simulink model "CSE1_Full"  (R2019a)
settings: Solver=VariableStepAuto  StartTime=0.0  StopTime=200  MaxStep=10e-3  RelTol=1e-3
values from neighbouring files (symbols this model uses):
  alpha1 = 0    [main.m]
  alpha2 = 3*pi/4    (= 2.35619449019)    [main.m]
  b = [0;0;0]    [main.m]
  C1 = pinv(B1*K1)    [main.m]
  C2 = inv(K2)*inv(B2)    [main.m]
  center = [0; 0]    [main.m]
  D = [d_11 0 0 ... (first row only)    [main.m]
  inv_M = inv(M)    [main.m]
  K_1 = 10*diag([2 2 2])    [main.m]
  K_2 = 10*diag([2 2 2])    [main.m]
  L_1 = diag([12 12 12])    [main.m]
  L_2 = diag([8 8 8])    [main.m]
  L_3 = diag([1 1 1])    [main.m]
  M = [m_11 0    0 ... (first row only)    [main.m]
  mu = 10e-4    (= 0.001)    [main.m]
  pd_final = [10;4]    [main.m]
  pd_initial = [0;0]    [main.m]
  R = [2; 3]    [main.m]
  Umax_1 = 0.1    [main.m]
  Umax_2 = 0.05    [main.m]
libraries: lib x9
settings Model: Creator=einarsu  LastModifiedBy=zhy
settings DataIOCC: ReturnWorkspaceOutputs=off
settings DebuggingCC: PregeneratedLibrarySubsystemCodeDiagnostic=none  SFExecutionAtInitializationDiag=none  ArithmeticOperatorsInVariantConditions=warning
settings HardwareCC: TargetBitPerPointer=64  TargetBitPerSizeT=64  TargetBitPerPtrDiffT=64  TargetLongLongMode=on  TargetIntDivRoundTo=Zero  TargetEndianess=LittleEndian  TargetWordSize=64  TargetHWDeviceType=MATLAB Host  ProdEqTarget=off
settings SFSimCC: SimUseLocalCustomCode=off
settings RTWCC: SystemTargetFile=rsim.tlc  TemplateMakefile=rsim_default_tmf  Description=Rapid Simulation Target  RTWUseLocalCustomCode=off
settings CodeAppCC: StateflowObjectComments=on
settings TargetCC: TargetLangStandard=C99 (ISO)  ParMdlRefBuildCompliant=on  ConcurrentExecutionCompliant=on  GeneratePreprocessorConditionals=Use local settings  MatFileLogging=on  PreserveStateflowLocalDataDimensions=off

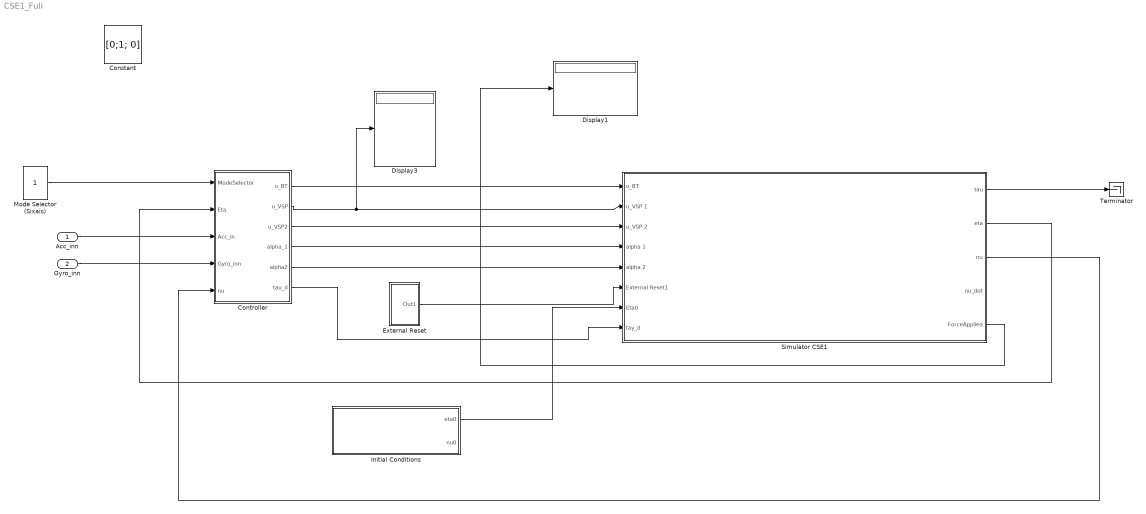
== system CSE1_Full ==
  Acc_inn : Inport
  Gyro_inn : Inport  Port=2
  Constant : Constant  Value=[0;1; 0]
  Controller : Subsystem
  Display1 : Display
  Display3 : Display
  External Reset : Subsystem
  "Initial Conditions " : Subsystem
  Mode Selector (Sixais) : Constant
  Simulator CSE1 : Subsystem
  Terminator : Terminator
  wires:
  Controller/1(u_BT) -> Simulator CSE1/1(u_BT)
  Controller/4(alpha_1) -> Simulator CSE1/4(alpha 1)
  Controller/2(u_VSP) -> Display3/1, Simulator CSE1/2(u_VSP 1)
  Controller/5(alpha2) -> Simulator CSE1/5(alpha 2)
  Controller/3("u_VSP2 ") -> Simulator CSE1/3(u_VSP 2)
  Simulator CSE1/1(tau) -> Terminator/1
  External Reset/1(Out1) -> Simulator CSE1/6(External Reset1)
  "Initial Conditions "/1(eta0) -> Simulator CSE1/7(Eta0)
  Mode Selector (Sixais)/1 -> Controller/1(ModeSelector)
  Simulator CSE1/2(eta) -> Controller/2(Eta)
  Acc_inn/1 -> Controller/3(Acc_in)
  Gyro_inn/1 -> Controller/4(Gyro_inn)
  Simulator CSE1/5(ForceApplied) -> Display1/1
  Simulator CSE1/3(nu) -> Controller/5("nu ")
  Controller/6(tau_d) -> Simulator CSE1/8(tay_d)

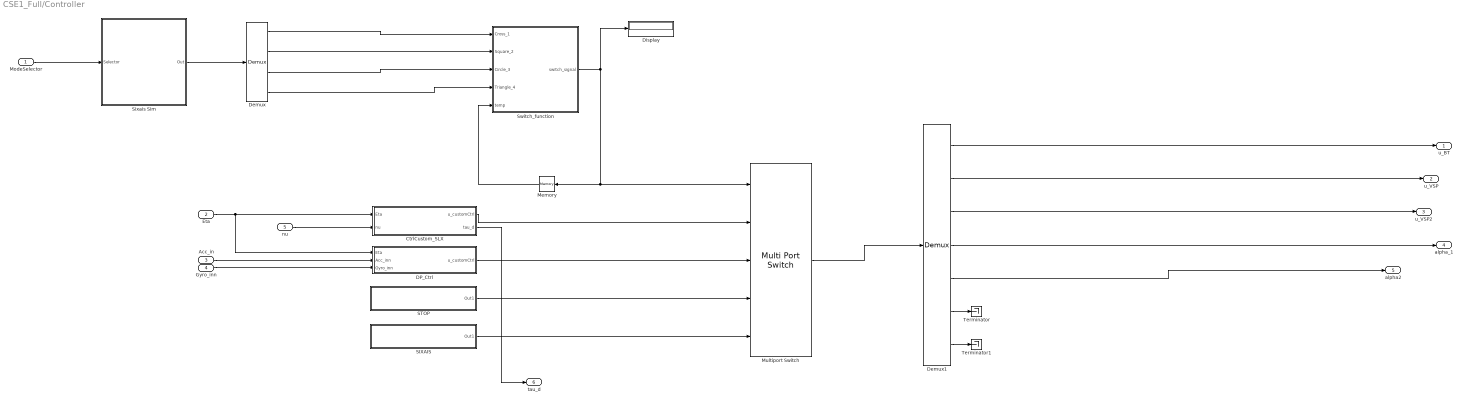
== system CSE1_Full/Controller ==
  ModeSelector : Inport
  Eta : Inport  Port=2
  Acc_in : Inport  Port=3
  Gyro_inn : Inport  Port=4
  "nu " : Inport  Port=5
  CtrlCustom_SLX : Subsystem
  DP_Ctrl : Subsystem
  Demux : Demux
  Demux1 : Demux  Outputs=7
  Display : Display
  Memory : Memory  InitialCondition=4
  Multiport Switch : MultiPortSwitch  Inputs=4
  SIXAIS : Subsystem
  STOP : Subsystem
  Sixais Sim : MATLAB Function  TreatAsAtomicUnit=on
  Switch_function : MATLAB Function  TreatAsAtomicUnit=on
  Terminator : Terminator
  Terminator1 : Terminator
  u_BT : Outport
  u_VSP : Outport  Port=2
  "u_VSP2 " : Outport  Port=3
  alpha_1 : Outport  Port=4
  alpha2 : Outport  Port=5
  tau_d : Outport  Port=6
  wires:
  Switch_function/1(switch_signal) -> Memory/1, Multiport Switch/1, Display/1
  Memory/1 -> Switch_function/5(temp)
  CtrlCustom_SLX/1(u_customCtrl) -> Multiport Switch/2
  Demux/1 -> Switch_function/1(Cross_1)
  Demux/2 -> Switch_function/2(Square_2)
  Demux/3 -> Switch_function/3(Circle_3)
  Demux/4 -> Switch_function/4(Triangle_4)
  Sixais Sim/1(Out) -> Demux/1
  ModeSelector/1 -> Sixais Sim/1(Selector)
  DP_Ctrl/1(u_customCtrl) -> Multiport Switch/3
  STOP/1(Out1) -> Multiport Switch/4
  SIXAIS/1(Out1) -> Multiport Switch/5
  Eta/1 -> CtrlCustom_SLX/1(Eta), DP_Ctrl/1(Eta)
  Acc_in/1 -> DP_Ctrl/2(Acc_inn)
  Gyro_inn/1 -> DP_Ctrl/3(Gyro_inn)
  Multiport Switch/1 -> Demux1/1
  Demux1/1 -> u_BT/1
  Demux1/2 -> u_VSP/1
  Demux1/3 -> "u_VSP2 "/1
  Demux1/4 -> alpha_1/1
  Demux1/5 -> alpha2/1
  Demux1/6 -> Terminator/1
  Demux1/7 -> Terminator1/1
  "nu "/1 -> CtrlCustom_SLX/2(nu)
  CtrlCustom_SLX/2(tau_d) -> tau_d/1

== system CSE1_Full/External Reset ==
  note: Most relevant for Real-Time Simulations...
  Constant : Constant  Value=0
  Out1 : Outport
  wires:
  Constant/1 -> Out1/1

== system CSE1_Full/Initial Conditions  ==
  Eta0 : Constant  Value=[0 0 0]
  "V0 " : Constant  Value=zeros(3,1)
  eta0 : Outport
  nu0 : Outport  Port=2
  wires:
  "V0 "/1 -> nu0/1
  Eta0/1 -> eta0/1

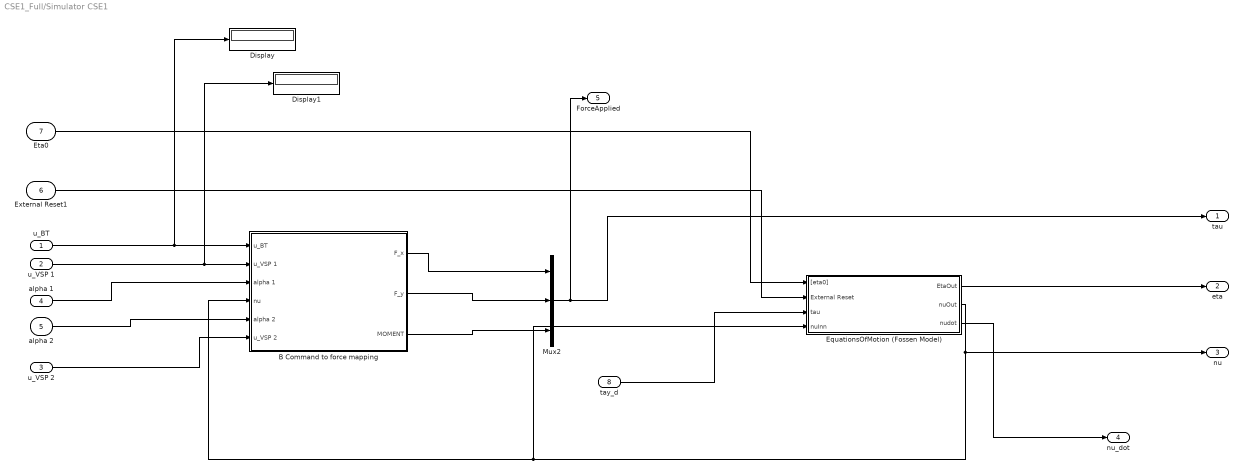
== system CSE1_Full/Simulator CSE1 ==
  u_BT : Inport
  u_VSP 1 : Inport  Port=2
  u_VSP 2 : Inport  Port=3
  alpha 1 : Inport  Port=4
  alpha 2 : Inport  Port=5
  External Reset1 : Inport  Port=6
  Eta0 : Inport  Port=7
  tay_d : Inport  Port=8
  B Command to force mapping : Subsystem
  Display : Display
  Display1 : Display
  EquationsOfMotion (Fossen Model) : Subsystem
  Mux2 : Mux  Inputs=3
  tau : Outport
  eta : Outport  Port=2
  nu : Outport  Port=3
  nu_dot : Outport  Port=4
  ForceApplied : Outport  Port=5
  wires:
  alpha 2/1 -> B Command to force mapping/5(alpha 2)
  B Command to force mapping/2("F_y ") -> Mux2/2
  B Command to force mapping/1(F_x) -> Mux2/1
  u_VSP 1/1 -> B Command to force mapping/2(u_VSP 1), Display1/1
  alpha 1/1 -> B Command to force mapping/3(alpha 1)
  u_BT/1 -> B Command to force mapping/1(u_BT), Display/1
  u_VSP 2/1 -> B Command to force mapping/6(u_VSP 2)
  Eta0/1 -> EquationsOfMotion (Fossen Model)/1("[eta0] ")
  External Reset1/1 -> EquationsOfMotion (Fossen Model)/2(External Reset)
  Mux2/1 -> ForceApplied/1, tau/1
  EquationsOfMotion (Fossen Model)/3(nudot) -> nu_dot/1
  B Command to force mapping/3("MOMENT ") -> Mux2/3
  EquationsOfMotion (Fossen Model)/1(EtaOut) -> eta/1
  EquationsOfMotion (Fossen Model)/2(nuOut) -> B Command to force mapping/4(nu), EquationsOfMotion (Fossen Model)/4(nuInn), nu/1
  tay_d/1 -> EquationsOfMotion (Fossen Model)/3(tau)

== system CSE1_Full/Controller/CtrlCustom_SLX ==
  Eta : Inport
  nu : Inport  Port=2
  Controller & Observor : Subsystem
  Pose : Subsystem
  Scope : Subsystem
  Selector : Selector  InputPortWidth=3  IndexOptions=Index vector (dialog)  Indices=[1 2]  OutputSizes=1
  Thrust Allocation : Subsystem
  To Workspace : ToWorkspace  VariableName=simout  SaveFormat=Structure With Time  SampleTime=-1
  u : Subsystem
  u_customCtrl : Outport
  tau_d : Outport  Port=2
  wires:
  u/1(u_out) -> u_customCtrl/1
  Eta/1 -> Pose/1(eta)
  Pose/1(QTM) -> Selector/1, Scope/3(eta), Controller & Observor/1(eta)
  nu/1 -> Scope/1(nu)
  Controller & Observor/1(nu_hat) -> Scope/2(nu_hat)
  Thrust Allocation/1(u) -> u/1(u)
  Controller & Observor/2(eta_hat) -> Scope/4(eta_hat)
  Controller & Observor/3(tau_d) -> tau_d/1, Thrust Allocation/1(tau_d)
  Selector/1 -> To Workspace/1

== system CSE1_Full/Controller/DP_Ctrl ==
  Eta : Inport
  Acc_inn : Inport  Port=2
  Gyro_inn : Inport  Port=3
  Constant : Constant  Value=[1;0;0]
  IMU (Consider if going to be properly Simulated...) : Subsystem
  Pose : Subsystem
  "Thrust Allocation " : Subsystem
  u : Subsystem
  u_customCtrl : Outport
  wires:
  Pose/1(QTM) -> ?
  Gyro_inn/1 -> IMU (Consider if going to be properly Simulated...)/1(Gyro_inn)
  Acc_inn/1 -> IMU (Consider if going to be properly Simulated...)/2(Acc_inn)
  Eta/1 -> Pose/1(eta)
  u/1(Out1) -> u_customCtrl/1
  IMU (Consider if going to be properly Simulated...)/2(Gyro) -> ?
  IMU (Consider if going to be properly Simulated...)/1(Acc) -> ?
  Constant/1 -> "Thrust Allocation "/1(In1)
  "Thrust Allocation "/1(Out1) -> ?

== system CSE1_Full/Controller/SIXAIS ==
  Constant{,1..6} (7 alike) : Constant  Value=0
  Sixais Controller Not Simulated in Simulink : Subsystem
  Out1 : Outport
  wires:
  Constant/1 -> Sixais Controller Not Simulated in Simulink/1(In1)
  Constant1/1 -> Sixais Controller Not Simulated in Simulink/2(In2)
  Constant2/1 -> Sixais Controller Not Simulated in Simulink/3(In3)
  Constant3/1 -> Sixais Controller Not Simulated in Simulink/4(In4)
  Constant4/1 -> Sixais Controller Not Simulated in Simulink/5(In5)
  Constant5/1 -> Sixais Controller Not Simulated in Simulink/6(In6)
  Constant6/1 -> Sixais Controller Not Simulated in Simulink/7(In7)
  Sixais Controller Not Simulated in Simulink/1(Out1) -> Out1/1

== system CSE1_Full/Controller/STOP ==
  Constant{,1..6} (7 alike) : Constant  Value=0
  Mux1 : Mux  Inputs=7
  Out1 : Outport
  wires:
  Mux1/1 -> Out1/1
  Constant/1 -> Mux1/1
  Constant1/1 -> Mux1/2
  Constant2/1 -> Mux1/3
  Constant3/1 -> Mux1/4
  Constant4/1 -> Mux1/5
  Constant5/1 -> Mux1/6
  Constant6/1 -> Mux1/7

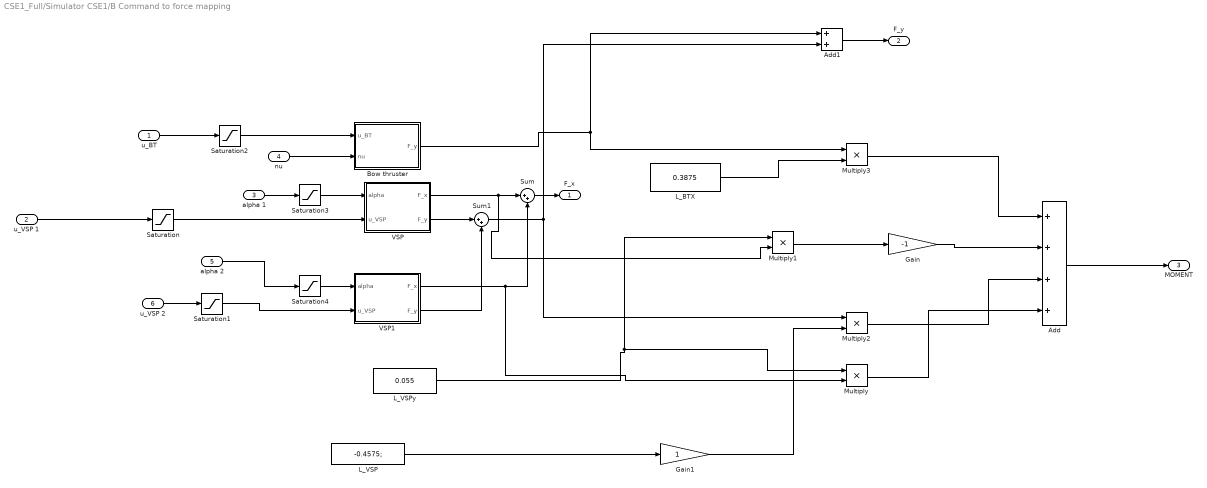
== system CSE1_Full/Simulator CSE1/B Command to force mapping ==
  u_BT : Inport
  u_VSP 1 : Inport  Port=2
  alpha 1 : Inport  Port=3
  nu : Inport  Port=4
  alpha 2 : Inport  Port=5
  u_VSP 2 : Inport  Port=6
  Add : Sum  Inputs=++++
  Add1 : Sum
  Bow thruster : MATLAB Function  TreatAsAtomicUnit=on
  Gain : Gain  Gain=-1
  Gain1 : Gain
  L_BTX : Constant  Value=0.3875
  L_VSP : Constant  Value=-0.4575;
  L_VSPy : Constant  Value=0.055
  Multiply{,1..3} (4 alike) : Product
  Saturation : Saturate  UpperLimit=1  LowerLimit=0
  Saturation1 : Saturate  UpperLimit=1  LowerLimit=0
  Saturation2 : Saturate  UpperLimit=1  LowerLimit=-1
  Saturation3 : Saturate  UpperLimit=pi  LowerLimit=-pi
  Saturation4 : Saturate  UpperLimit=pi  LowerLimit=-pi
  Sum : Sum  Inputs=|++
  Sum1 : Sum  Inputs=|++
  VSP : MATLAB Function  TreatAsAtomicUnit=on
  VSP1 : MATLAB Function  TreatAsAtomicUnit=on
  F_x : Outport
  "F_y " : Outport  Port=2
  "MOMENT " : Outport  Port=3
  wires:
  alpha 1/1 -> Saturation3/1
  nu/1 -> Bow thruster/2(nu)
  Bow thruster/1(F_y) -> Add1/1, Multiply3/1
  VSP/2(F_y) -> Sum1/1
  Sum1/1 -> Add1/2, Multiply2/1
  VSP1/2(F_y) -> Sum1/2
  VSP1/1(F_x) -> Multiply/2, Sum/2
  VSP/1(F_x) -> Multiply1/2, Sum/1
  Sum/1 -> F_x/1
  alpha 2/1 -> Saturation4/1
  u_VSP 2/1 -> Saturation1/1
  L_VSP/1 -> Gain1/1
  L_BTX/1 -> Multiply3/2
  L_VSPy/1 -> Multiply/1, Multiply1/1
  Multiply3/1 -> Add/1
  Multiply1/1 -> Gain/1
  Multiply2/1 -> Add/3
  Multiply/1 -> Add/4
  Add/1 -> "MOMENT "/1
  Gain/1 -> Add/2
  Gain1/1 -> Multiply2/2
  Add1/1 -> "F_y "/1
  Saturation/1 -> VSP/2(u_VSP)
  Saturation1/1 -> VSP1/2(u_VSP)
  u_BT/1 -> Saturation2/1
  u_VSP 1/1 -> Saturation/1
  Saturation2/1 -> Bow thruster/1(u_BT)
  Saturation3/1 -> VSP/1(alpha)
  Saturation4/1 -> VSP1/1(alpha)

== system CSE1_Full/Simulator CSE1/EquationsOfMotion (Fossen Model) ==
  "[eta0] " : Inport
  External Reset : Inport  Port=2
  tau : Inport  Port=3
  nuInn : Inport  Port=4
  Position : Integrator  ExternalReset=either  InitialConditionSource=external  InitialCondition=[0 0 0]'
  Velocity : Integrator  ExternalReset=either  InitialCondition=[0 0 0]'
  kinematics : MATLAB Function  TreatAsAtomicUnit=on
  kinetics : MATLAB Function  TreatAsAtomicUnit=on
  EtaOut : Outport
  nuOut : Outport  Port=2
  nudot : Outport  Port=3
  wires:
  tau/1 -> kinetics/1(tau)
  Position/1 -> kinematics/2(eta), EtaOut/1
  "[eta0] "/1 -> Position/3
  nuInn/1 -> kinetics/2(nu)
  kinematics/1(eta_dot) -> Position/1
  Velocity/1 -> nuOut/1, kinematics/1(nu)
  kinetics/1(nu_dot) -> nudot/1, Velocity/1
  External Reset/1 -> Velocity/2, Position/2

== system CSE1_Full/Controller/CtrlCustom_SLX/Controller & Observor ==
  eta : Inport
  Controller : Subsystem
  Observer : Subsystem
  Update law : Subsystem
  nu_hat : Outport
  eta_hat : Outport  Port=2
  tau_d : Outport  Port=3
  Us_line : Outport  Port=4
  Us_ellipsoid : Outport  Port=5
  wires:
  eta/1 -> Update law/1(eta), Observer/1(eta)
  Observer/2(nu_hat) -> nu_hat/1, Controller/2(nu_hat)
  Observer/1(eta_hat) -> eta_hat/1, Controller/1(eta_hat)
  Controller/1(tau_d) -> Observer/2(tau_d), tau_d/1
  Update law/1(Us_line) -> Us_line/1
  Update law/2(eta_d) -> Controller/3(eta_d)
  Update law/3(eta_d_dot) -> Controller/4(eta_d_dot)
  Update law/4(eta_d_dot2) -> Controller/5(eta_d_dot2)
  Update law/5(Us_ellipsoid) -> Us_ellipsoid/1

== system CSE1_Full/Controller/CtrlCustom_SLX/Pose ==
  eta : Inport
  Demux : Demux  Outputs=3
  MATLAB Function : MATLAB Function  TreatAsAtomicUnit=on
  Mux : Mux  Inputs=3
  QTM : Outport
  wires:
  Demux/2 -> Mux/2  "y_m"
  Demux/1 -> Mux/1  "x_m"
  Mux/1 -> QTM/1
  eta/1 -> Demux/1
  Demux/3 -> Mux/3  "psi_m"

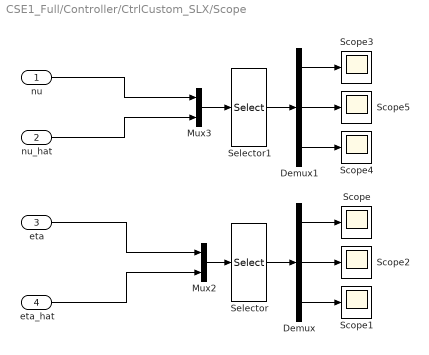
== system CSE1_Full/Controller/CtrlCustom_SLX/Scope ==
  nu : Inport
  nu_hat : Inport  Port=2
  eta : Inport  Port=3
  eta_hat : Inport  Port=4
  Demux : Demux  Outputs=3
  Demux1 : Demux  Outputs=3
  Mux2 : Mux  Inputs=2
  Mux3 : Mux  Inputs=2
  Scope{,1..5} (6 alike) : Scope
  Selector : Selector  InputPortWidth=6  IndexOptions=Index vector (dialog)  Indices=[1 4 2 5 3 6]  OutputSizes=1
  Selector1 : Selector  InputPortWidth=6  IndexOptions=Index vector (dialog)  Indices=[1 4 2 5 3 6]  OutputSizes=1
  wires:
  Selector/1 -> Demux/1
  Demux/1 -> Scope/1
  Demux/3 -> Scope1/1
  Demux1/1 -> Scope3/1
  Demux1/3 -> Scope4/1
  Demux1/2 -> Scope5/1
  Mux2/1 -> Selector/1
  Mux3/1 -> Selector1/1
  Demux/2 -> Scope2/1
  nu_hat/1 -> Mux3/2
  Selector1/1 -> Demux1/1
  nu/1 -> Mux3/1
  eta/1 -> Mux2/1
  eta_hat/1 -> Mux2/2

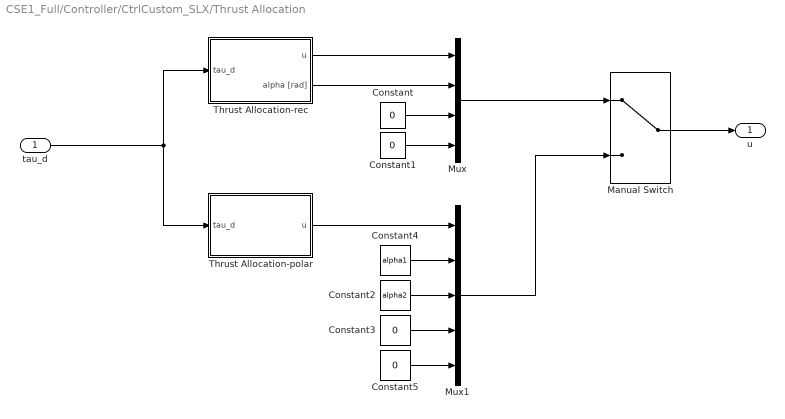
== system CSE1_Full/Controller/CtrlCustom_SLX/Thrust Allocation ==
  tau_d : Inport
  Constant{,1,3,5} (4 alike) : Constant  Value=0
  Constant2 : Constant  Value=alpha2
  Constant4 : Constant  Value=alpha1
  Manual Switch : ManualSwitch
  Mux : Mux
  Mux1 : Mux  Inputs=5
  Thrust Allocation-polar : Subsystem
  Thrust Allocation-rec : Subsystem
  u : Outport
  wires:
  tau_d/1 -> Thrust Allocation-polar/1(tau_d), Thrust Allocation-rec/1(tau_d)
  Thrust Allocation-rec/1(u) -> Mux/1
  Thrust Allocation-polar/1(u) -> Mux1/1
  Constant3/1 -> Mux1/4
  Constant4/1 -> Mux1/2
  Mux/1 -> Manual Switch/1
  Mux1/1 -> Manual Switch/2
  Constant2/1 -> Mux1/3
  Constant5/1 -> Mux1/5
  Constant/1 -> Mux/3
  Thrust Allocation-rec/2(alpha [rad]) -> Mux/2
  Constant1/1 -> Mux/4
  Manual Switch/1 -> u/1

== system CSE1_Full/Controller/CtrlCustom_SLX/u ==
  u : Inport
  Demux1 : Demux  Outputs=7
  Mux : Mux  Inputs=7
  Saturation1 : Saturate  UpperLimit=1  LowerLimit=0
  Saturation11 : Saturate  UpperLimit=1  LowerLimit=0
  u_out : Outport
  wires:
  u/1 -> Demux1/1
  Demux1/1 -> Mux/1  "u_BT"
  Demux1/2 -> Saturation11/1  "u_VSP1"
  Demux1/3 -> Saturation1/1  "u_VSP2"
  Demux1/4 -> Mux/4  "alpha_VSP1"
  Demux1/5 -> Mux/5  "alpha_VSP2"
  Demux1/6 -> Mux/6  "omega_VSP1"
  Demux1/7 -> Mux/7  "omega_VSP2"
  Mux/1 -> u_out/1
  Saturation11/1 -> Mux/2
  Saturation1/1 -> Mux/3

== system CSE1_Full/Controller/DP_Ctrl/IMU (Consider if going to be properly Simulated...) ==
  Gyro_inn : Inport
  Acc_inn : Inport  Port=2
  Demux : Demux  Outputs=3
  Demux1 : Demux  Outputs=3
  Mux : Mux  Inputs=3
  Mux2 : Mux  Inputs=3
  Acc : Outport
  Gyro : Outport  Port=2
  wires:
  Acc_inn/1 -> Demux1/1
  Gyro_inn/1 -> Demux/1
  Demux/1 -> Mux2/1
  Demux/2 -> Mux2/2
  Demux/3 -> Mux2/3
  Demux1/2 -> Mux/2
  Demux1/3 -> Mux/3
  Mux2/1 -> Gyro/1
  Demux1/1 -> Mux/1
  Mux/1 -> Acc/1

== system CSE1_Full/Controller/DP_Ctrl/Pose ==
  eta : Inport
  Demux : Demux  Outputs=3
  Mux : Mux  Inputs=3
  QTM : Outport
  wires:
  eta/1 -> Demux/1
  Mux/1 -> QTM/1
  Demux/1 -> Mux/1  "x_m"
  Demux/3 -> Mux/3  "psi_m"
  Demux/2 -> Mux/2  "y_m"

== system CSE1_Full/Controller/DP_Ctrl/Thrust Allocation  ==
  In1 : Inport
  THALOC (u->tau) : MATLAB Function  TreatAsAtomicUnit=on
  Out1 : Outport
  wires:
  In1/1 -> THALOC (u->tau)/1(u)
  THALOC (u->tau)/1(y) -> Out1/1

== system CSE1_Full/Controller/DP_Ctrl/u ==
  In1 : Inport
  Demux1 : Demux  Outputs=7
  Mux : Mux  Inputs=7
  Out1 : Outport
  wires:
  Mux/1 -> Out1/1
  Demux1/7 -> Mux/7  "omega_VSP2"
  Demux1/6 -> Mux/6  "omega_VSP1"
  Demux1/5 -> Mux/5  "alpha_VSP2"
  Demux1/4 -> Mux/4  "alpha_VSP1"
  Demux1/3 -> Mux/3  "u_VSP2"
  Demux1/2 -> Mux/2  "u_VSP1"
  Demux1/1 -> Mux/1  "u_BT"
  In1/1 -> Demux1/1

== system CSE1_Full/Controller/SIXAIS/Sixais Controller Not Simulated in Simulink ==
  In1 : Inport
  In2 : Inport  Port=2
  In3 : Inport  Port=3
  In4 : Inport  Port=4
  In5 : Inport  Port=5
  In6 : Inport  Port=6
  In7 : Inport  Port=7
  Mux1 : Mux  Inputs=7
  Out1 : Outport
  wires:
  In4/1 -> Mux1/4
  In5/1 -> Mux1/5
  In6/1 -> Mux1/6
  In3/1 -> Mux1/3
  In1/1 -> Mux1/1
  In2/1 -> Mux1/2
  Mux1/1 -> Out1/1
  In7/1 -> Mux1/7

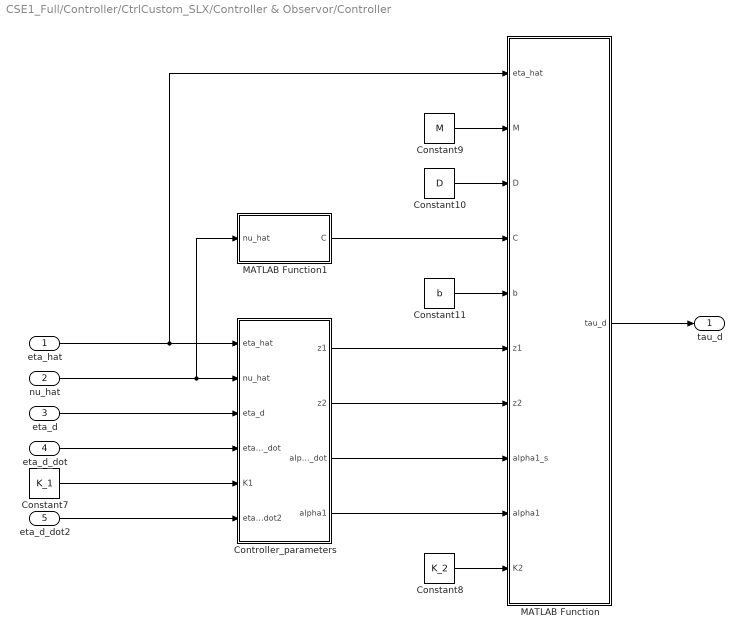
== system CSE1_Full/Controller/CtrlCustom_SLX/Controller & Observor/Controller ==
  eta_hat : Inport
  nu_hat : Inport  Port=2
  eta_d : Inport  Port=3
  eta_d_dot : Inport  Port=4
  eta_d_dot2 : Inport  Port=5
  Constant10 : Constant  Value=D
  Constant11 : Constant  Value=b
  Constant7 : Constant  Value=K_1
  Constant8 : Constant  Value=K_2
  Constant9 : Constant  Value=M
  Controller_parameters : Subsystem
  MATLAB Function : MATLAB Function  TreatAsAtomicUnit=on
  MATLAB Function1 : MATLAB Function  TreatAsAtomicUnit=on
  tau_d : Outport
  wires:
  Controller_parameters/4(alpha1) -> MATLAB Function/9(alpha1)
  nu_hat/1 -> MATLAB Function1/1(nu_hat), Controller_parameters/2(nu_hat)
  Controller_parameters/2(z2) -> MATLAB Function/7(z2)
  Constant7/1 -> Controller_parameters/5(K1)
  Constant10/1 -> MATLAB Function/3(D)
  Constant9/1 -> MATLAB Function/2(M)
  Constant11/1 -> MATLAB Function/5(b)
  eta_d_dot/1 -> Controller_parameters/4(eta_d_dot)
  Constant8/1 -> MATLAB Function/10(K2)
  Controller_parameters/1(z1) -> MATLAB Function/6(z1)
  Controller_parameters/3(alpha1_dot) -> MATLAB Function/8(alpha1_s)
  eta_d/1 -> Controller_parameters/3(eta_d)
  eta_hat/1 -> MATLAB Function/1(eta_hat), Controller_parameters/1(eta_hat)
  eta_d_dot2/1 -> Controller_parameters/6(eta_d_dot2)
  MATLAB Function/1(tau_d) -> tau_d/1
  MATLAB Function1/1(C) -> MATLAB Function/4(C)

== system CSE1_Full/Controller/CtrlCustom_SLX/Controller & Observor/Observer ==
  eta : Inport
  tau_d : Inport  Port=2
  Demux : Demux  Outputs=2
  Manual Switch : ManualSwitch
  Mux : Mux  Inputs=2
  Mux1 : Mux  Inputs=2
  Obs with bias : Subsystem
  Obs without bias : Subsystem
  eta_hat : Outport
  nu_hat : Outport  Port=2
  wires:
  eta/1 -> Obs without bias/1(eta), Obs with bias/1(eta)
  tau_d/1 -> Obs with bias/2(tau_d), Obs without bias/2(tau_d)
  Obs without bias/1(nu_hat) -> Mux1/1
  Obs without bias/2(eta_hat) -> Mux1/2
  Obs with bias/1(nu_hat) -> Mux/1
  Obs with bias/2(eta_hat) -> Mux/2
  Mux/1 -> Manual Switch/1
  Mux1/1 -> Manual Switch/2
  Manual Switch/1 -> Demux/1
  Demux/2 -> eta_hat/1
  Demux/1 -> nu_hat/1

== system CSE1_Full/Controller/CtrlCustom_SLX/Controller & Observor/Update law ==
  eta : Inport
  Manual Switch1 : ManualSwitch
  Manual Switch2 : ManualSwitch
  Manual Switch4 : ManualSwitch
  ellipsoid : Subsystem
  straight line : Subsystem
  Us_line : Outport
  eta_d : Outport  Port=2
  eta_d_dot : Outport  Port=3
  eta_d_dot2 : Outport  Port=4
  Us_ellipsoid : Outport  Port=5
  wires:
  ellipsoid/3(Us) -> Us_ellipsoid/1
  straight line/3(Us) -> Us_line/1
  straight line/2(eta_d_dot) -> Manual Switch2/1
  ellipsoid/4(eta_d_dot2) -> Manual Switch4/2
  Manual Switch1/1 -> eta_d/1
  eta/1 -> straight line/1(eta), ellipsoid/1(eta)
  straight line/1(eta_d) -> Manual Switch1/1
  straight line/4(eta_d_dot2) -> Manual Switch4/1
  ellipsoid/2(eta_d_dot) -> Manual Switch2/2
  ellipsoid/1(eta_d) -> Manual Switch1/2
  Manual Switch2/1 -> eta_d_dot/1
  Manual Switch4/1 -> eta_d_dot2/1

== system CSE1_Full/Controller/CtrlCustom_SLX/Thrust Allocation/Thrust Allocation-polar ==
  tau_d : Inport
  Gain : Gain  Gain=C2  Multiplication=Matrix(K*u)
  u : Outport
  wires:
  tau_d/1 -> Gain/1
  Gain/1 -> u/1

== system CSE1_Full/Controller/CtrlCustom_SLX/Thrust Allocation/Thrust Allocation-rec ==
  tau_d : Inport
  Demux : Demux  Outputs=5
  Gain : Gain  Gain=C1  Multiplication=Matrix(K*u)
  Mux : Mux  Inputs=2
  Mux2 : Mux  Inputs=3
  VSP1 : Subsystem
  VSP2 : Subsystem
  u : Outport
  alpha [rad] : Outport  Port=2
  wires:
  Mux/1 -> alpha [rad]/1
  Gain/1 -> Demux/1
  Mux2/1 -> u/1
  tau_d/1 -> Gain/1
  VSP1/2(Alpha_1) -> Mux/1
  VSP2/2(Alpha_2) -> Mux/2
  Demux/1 -> VSP1/1(u_1x)
  Demux/2 -> VSP1/2(u_1y)
  Demux/3 -> VSP2/1(u_2x)
  Demux/4 -> VSP2/2(u_2y)
  VSP2/1(u_2) -> Mux2/2
  VSP1/1(u_1) -> Mux2/1
  Demux/5 -> Mux2/3

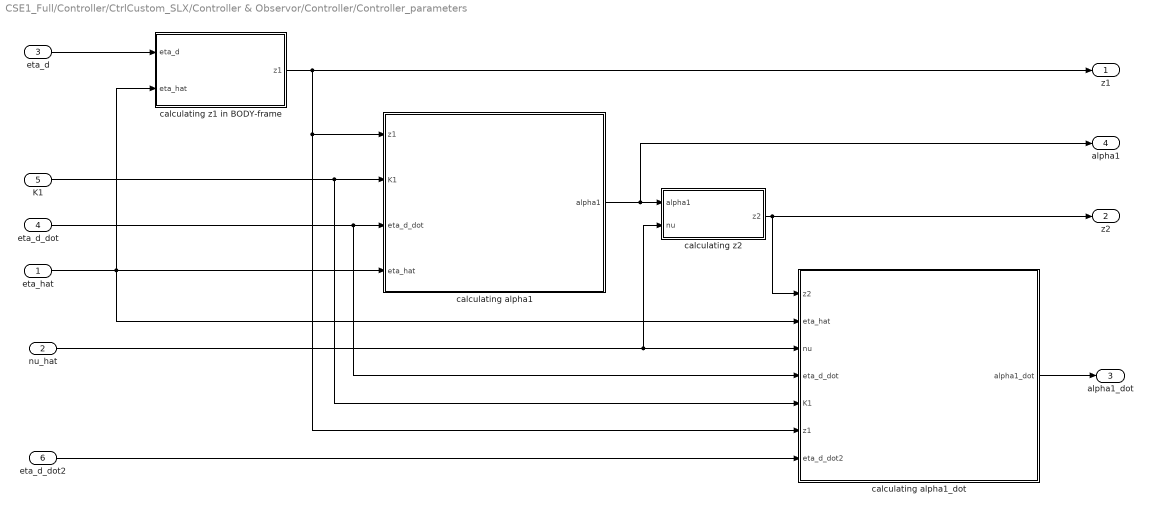
== system CSE1_Full/Controller/CtrlCustom_SLX/Controller & Observor/Controller/Controller_parameters ==
  eta_hat : Inport
  nu_hat : Inport  Port=2
  eta_d : Inport  Port=3
  eta_d_dot : Inport  Port=4
  K1 : Inport  Port=5
  eta_d_dot2 : Inport  Port=6
  calculating alpha1 : MATLAB Function  TreatAsAtomicUnit=on
  calculating alpha1_dot : MATLAB Function  TreatAsAtomicUnit=on
  calculating z1 in BODY-frame : MATLAB Function  TreatAsAtomicUnit=on
  calculating z2 : MATLAB Function  TreatAsAtomicUnit=on
  z1 : Outport
  z2 : Outport  Port=2
  alpha1_dot : Outport  Port=3
  alpha1 : Outport  Port=4
  wires:
  eta_hat/1 -> calculating alpha1_dot/2(eta_hat), calculating z1 in BODY-frame/2(eta_hat), calculating alpha1/4(eta_hat)
  eta_d/1 -> calculating z1 in BODY-frame/1(eta_d)
  eta_d_dot/1 -> calculating alpha1/3(eta_d_dot), calculating alpha1_dot/4(eta_d_dot)
  nu_hat/1 -> calculating z2/2(nu), calculating alpha1_dot/3(nu)
  calculating alpha1_dot/1(alpha1_dot) -> alpha1_dot/1
  calculating alpha1/1(alpha1) -> alpha1/1, calculating z2/1(alpha1)
  K1/1 -> calculating alpha1_dot/5(K1), calculating alpha1/2(K1)
  calculating z2/1(z2) -> z2/1, calculating alpha1_dot/1(z2)
  calculating z1 in BODY-frame/1(z1) -> calculating alpha1_dot/6(z1), calculating alpha1/1(z1), z1/1
  eta_d_dot2/1 -> calculating alpha1_dot/7(eta_d_dot2)

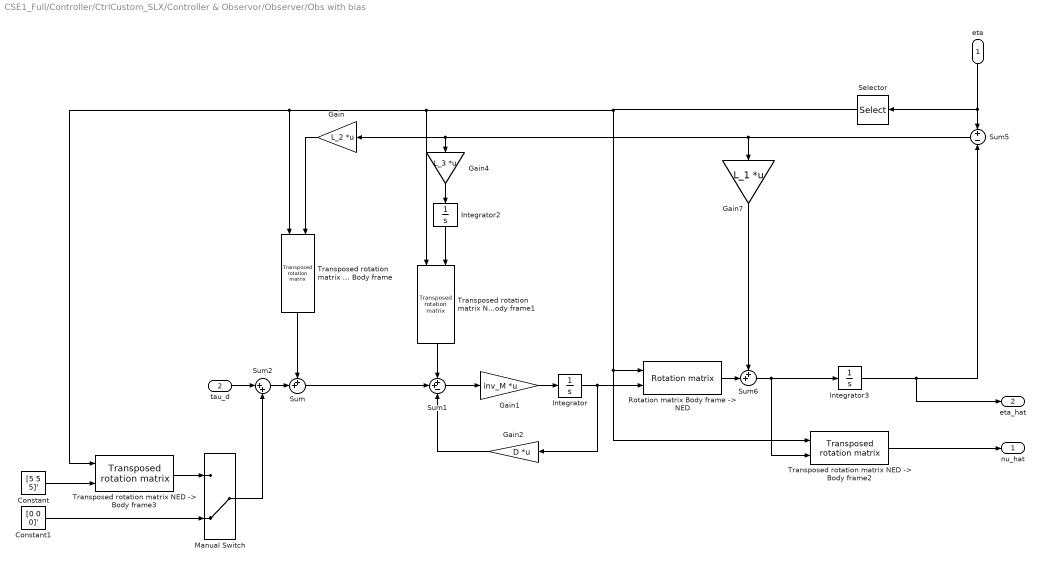
== system CSE1_Full/Controller/CtrlCustom_SLX/Controller & Observor/Observer/Obs with bias ==
  eta : Inport
  tau_d : Inport  Port=2
  Constant : Constant  Value=[5 5 5]'
  Constant1 : Constant  Value=[0 0 0]'
  Gain : Gain  Gain=L_2  Multiplication=Matrix(K*u)
  Gain1 : Gain  Gain=inv_M  Multiplication=Matrix(K*u)
  Gain2 : Gain  Gain=D  Multiplication=Matrix(K*u)
  Gain4 : Gain  Gain=L_3  Multiplication=Matrix(K*u)
  Gain7 : Gain  Gain=L_1  Multiplication=Matrix(K*u)
  Integrator : Integrator
  Integrator2 : Integrator
  Integrator3 : Integrator
  Manual Switch : ManualSwitch  CurrentSetting=0
  "Rotation matrix Body frame -> NED" : lib/Rotation matrix  SystemSampleTime=-1
  Selector : Selector  InputPortWidth=3  IndexOptions=Index vector (dialog)  Indices=[ 3]  OutputSizes=1
  Sum : Sum  Inputs=++|
  Sum1 : Sum  Inputs=++-
  Sum2 : Sum  Inputs=|++
  Sum5 : Sum  Inputs=+|-
  Sum6 : Sum  Inputs=++|
  Transposed rotation matrix NED -> Body frame{,1..3} (4 alike) : lib/Transposed rotation matrix  SystemSampleTime=-1
  nu_hat : Outport
  eta_hat : Outport  Port=2
  wires:
  Gain/1 -> "Transposed rotation matrix NED -> Body frame"/2
  "Transposed rotation matrix NED -> Body frame"/1 -> Sum/1
  "Transposed rotation matrix NED -> Body frame1"/1 -> Sum1/1
  Gain1/1 -> Integrator/1
  Integrator/1 -> Gain2/1, "Rotation matrix Body frame -> NED"/2
  "Rotation matrix Body frame -> NED"/1 -> Sum6/2
  Sum6/1 -> "Transposed rotation matrix NED -> Body frame2"/2, Integrator3/1
  Gain2/1 -> Sum1/3
  Sum/1 -> Sum1/2
  Integrator2/1 -> "Transposed rotation matrix NED -> Body frame1"/2
  Gain4/1 -> Integrator2/1
  Gain7/1 -> Sum6/1
  Sum1/1 -> Gain1/1
  eta/1 -> Selector/1, Sum5/1
  "Transposed rotation matrix NED -> Body frame2"/1 -> nu_hat/1
  Integrator3/1 -> Sum5/2, eta_hat/1
  Sum5/1 -> Gain4/1, Gain/1, Gain7/1
  Selector/1 -> "Transposed rotation matrix NED -> Body frame2"/1, "Rotation matrix Body frame -> NED"/1, "Transposed rotation matrix NED -> Body frame"/1, "Transposed rotation matrix NED -> Body frame3"/1, "Transposed rotation matrix NED -> Body frame1"/1
  "Transposed rotation matrix NED -> Body frame3"/1 -> Manual Switch/1
  Constant/1 -> "Transposed rotation matrix NED -> Body frame3"/2
  Constant1/1 -> Manual Switch/2
  Sum2/1 -> Sum/2
  tau_d/1 -> Sum2/1
  Manual Switch/1 -> Sum2/2

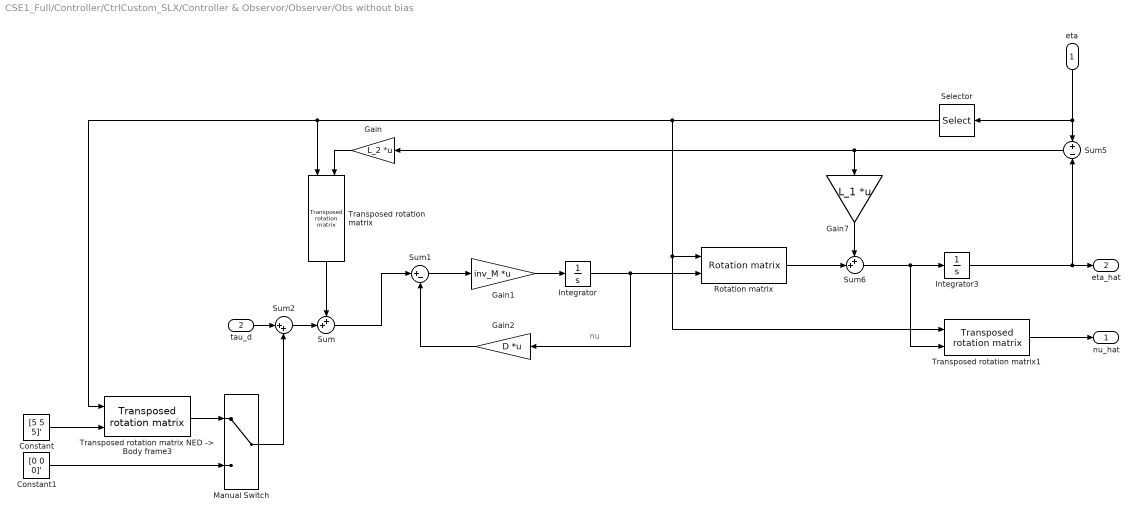
== system CSE1_Full/Controller/CtrlCustom_SLX/Controller & Observor/Observer/Obs without bias ==
  note: nu
  eta : Inport
  tau_d : Inport  Port=2
  Constant : Constant  Value=[5 5 5]'
  Constant1 : Constant  Value=[0 0 0]'
  Gain : Gain  Gain=L_2  Multiplication=Matrix(K*u)
  Gain1 : Gain  Gain=inv_M  Multiplication=Matrix(K*u)
  Gain2 : Gain  Gain=D  Multiplication=Matrix(K*u)
  Gain7 : Gain  Gain=L_1  Multiplication=Matrix(K*u)
  Integrator : Integrator
  Integrator3 : Integrator
  Manual Switch : ManualSwitch
  Rotation matrix : lib/Rotation matrix  SystemSampleTime=-1
  Selector : Selector  InputPortWidth=3  IndexOptions=Index vector (dialog)  Indices=[ 3]  OutputSizes=1
  Sum : Sum  Inputs=++|
  Sum1 : Sum  Inputs=|+-
  Sum2 : Sum  Inputs=|++
  Sum5 : Sum  Inputs=+|-
  Sum6 : Sum  Inputs=++|
  Transposed rotation matrix : lib/Transposed rotation matrix  SystemSampleTime=-1
  "Transposed rotation matrix NED -> Body frame3" : lib/Transposed rotation matrix  SystemSampleTime=-1
  Transposed rotation matrix1 : lib/Transposed rotation matrix  SystemSampleTime=-1
  nu_hat : Outport
  eta_hat : Outport  Port=2
  wires:
  Sum/1 -> Sum1/1
  Sum6/1 -> Transposed rotation matrix1/2, Integrator3/1
  Transposed rotation matrix1/1 -> nu_hat/1
  Gain7/1 -> Sum6/1
  Rotation matrix/1 -> Sum6/2
  Sum5/1 -> Gain/1, Gain7/1
  Gain1/1 -> Integrator/1
  Integrator3/1 -> Sum5/2, eta_hat/1
  Gain/1 -> Transposed rotation matrix/2
  Transposed rotation matrix/1 -> Sum/1
  Sum1/1 -> Gain1/1
  eta/1 -> Selector/1, Sum5/1
  Gain2/1 -> Sum1/2
  Integrator/1 -> Gain2/1, Rotation matrix/2
  Constant/1 -> "Transposed rotation matrix NED -> Body frame3"/2
  Selector/1 -> "Transposed rotation matrix NED -> Body frame3"/1, Transposed rotation matrix/1, Transposed rotation matrix1/1, Rotation matrix/1
  "Transposed rotation matrix NED -> Body frame3"/1 -> Manual Switch/1
  Manual Switch/1 -> Sum2/2
  Constant1/1 -> Manual Switch/2
  tau_d/1 -> Sum2/1
  Sum2/1 -> Sum/2

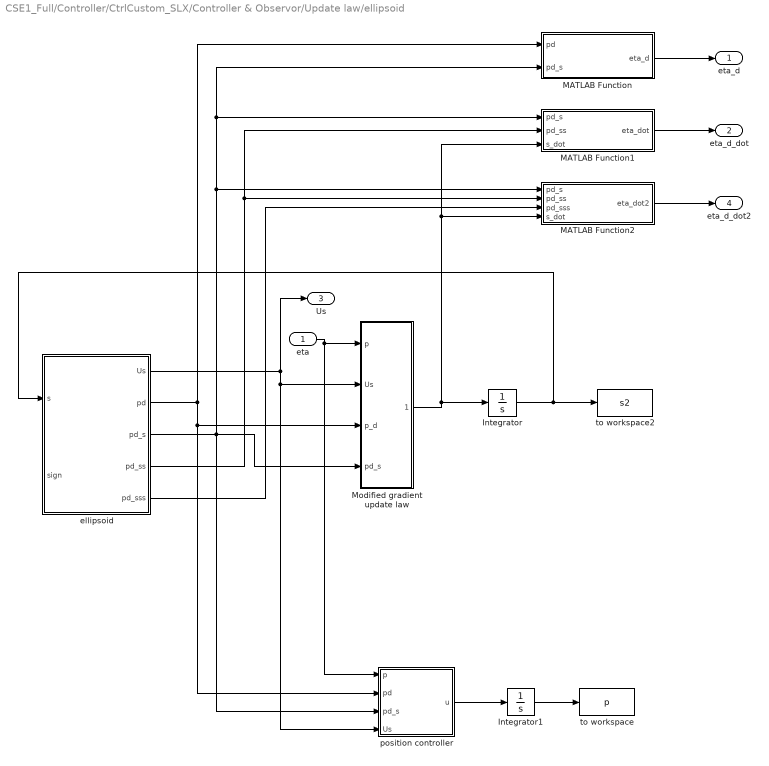
== system CSE1_Full/Controller/CtrlCustom_SLX/Controller & Observor/Update law/ellipsoid ==
  eta : Inport
  " Modified gradient update law" : Subsystem
  Integrator : Integrator
  Integrator1 : Integrator
  MATLAB Function : MATLAB Function  TreatAsAtomicUnit=on
  MATLAB Function1 : MATLAB Function  TreatAsAtomicUnit=on
  MATLAB Function2 : MATLAB Function  TreatAsAtomicUnit=on
  ellipsoid : Subsystem
  position controller : Subsystem
  to workspace : ToWorkspace  VariableName=p  SaveFormat=Timeseries  SampleTime=-1
  to workspace2 : ToWorkspace  VariableName=s2  SaveFormat=Timeseries  SampleTime=-1
  eta_d : Outport
  eta_d_dot : Outport  Port=2
  Us : Outport  Port=3
  eta_d_dot2 : Outport  Port=4
  wires:
  ellipsoid/1(Us) -> position controller/4(Us), " Modified gradient update law"/2(Us), Us/1
  ellipsoid/2(pd) -> position controller/2(pd), " Modified gradient update law"/3(p_d), MATLAB Function/1(pd)
  ellipsoid/3(pd_s) -> position controller/3(pd_s), MATLAB Function/2(pd_s), MATLAB Function1/1(pd_s), MATLAB Function2/1(pd_s), " Modified gradient update law"/4(pd_s)
  " Modified gradient update law"/1(s_dot) -> MATLAB Function2/4(s_dot), MATLAB Function1/3(s_dot), Integrator/1
  Integrator/1 -> ellipsoid/1(s), to workspace2/1
  eta/1 -> position controller/1(p), " Modified gradient update law"/1(p)
  MATLAB Function/1(eta_d) -> eta_d/1
  MATLAB Function1/1(eta_dot) -> eta_d_dot/1
  MATLAB Function2/1(eta_dot2) -> eta_d_dot2/1
  ellipsoid/4(pd_ss) -> MATLAB Function1/2(pd_ss), MATLAB Function2/2(pd_ss)
  ellipsoid/5(pd_sss) -> MATLAB Function2/3(pd_sss)
  position controller/1(u) -> Integrator1/1
  Integrator1/1 -> to workspace/1

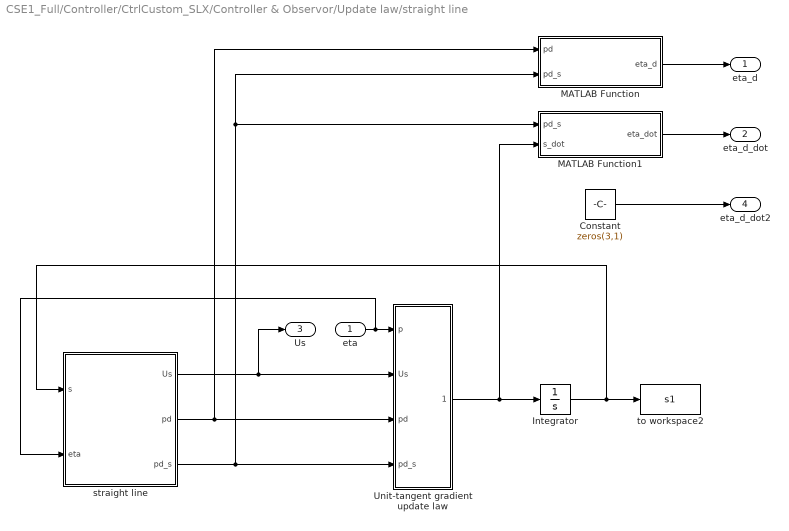
== system CSE1_Full/Controller/CtrlCustom_SLX/Controller & Observor/Update law/straight line ==
  eta : Inport
  Constant : Constant  Value=zeros(3,1)
  Integrator : Integrator
  MATLAB Function : MATLAB Function  TreatAsAtomicUnit=on
  MATLAB Function1 : MATLAB Function  TreatAsAtomicUnit=on
  Unit-tangent gradient update law : Subsystem
  straight line : Subsystem
  to workspace2 : ToWorkspace  VariableName=s1  SaveFormat=Timeseries  SampleTime=-1
  eta_d : Outport
  eta_d_dot : Outport  Port=2
  Us : Outport  Port=3
  eta_d_dot2 : Outport  Port=4
  wires:
  straight line/1(Us) -> Us/1, Unit-tangent gradient update law/2(Us)
  straight line/2(pd) -> MATLAB Function/1(pd), Unit-tangent gradient update law/3(pd)
  straight line/3(pd_s) -> MATLAB Function1/1(pd_s), MATLAB Function/2(pd_s), Unit-tangent gradient update law/4(pd_s)
  Unit-tangent gradient update law/1(s_dot) -> Integrator/1, MATLAB Function1/2(s_dot)
  Integrator/1 -> straight line/1(s), to workspace2/1
  eta/1 -> straight line/2(eta), Unit-tangent gradient update law/1(p)
  MATLAB Function/1(eta_d) -> eta_d/1
  MATLAB Function1/1(eta_dot) -> eta_d_dot/1
  Constant/1 -> eta_d_dot2/1

== system CSE1_Full/Controller/CtrlCustom_SLX/Thrust Allocation/Thrust Allocation-rec/VSP1 ==
  u_1x : Inport
  u_1y : Inport  Port=2
  Atan2 : Trigonometry  Operator=atan2
  Sqrt : Sqrt  SaturateOnIntegerOverflow=on
  Square : Math  Operator=square  SaturateOnIntegerOverflow=on
  Square1 : Math  Operator=square  SaturateOnIntegerOverflow=on
  Sum : Sum  Inputs=|++
  u_1 : Outport
  Alpha_1 : Outport  Port=2
  wires:
  u_1x/1 -> Atan2/2, Square/1
  u_1y/1 -> Square1/1, Atan2/1
  Square/1 -> Sum/1
  Square1/1 -> Sum/2
  Sum/1 -> Sqrt/1
  Sqrt/1 -> u_1/1
  Atan2/1 -> Alpha_1/1

== system CSE1_Full/Controller/CtrlCustom_SLX/Thrust Allocation/Thrust Allocation-rec/VSP2 ==
  u_2x : Inport
  u_2y : Inport  Port=2
  Atan2 : Trigonometry  Operator=atan2
  Sqrt : Sqrt  SaturateOnIntegerOverflow=on
  Square : Math  Operator=square  SaturateOnIntegerOverflow=on
  Square1 : Math  Operator=square  SaturateOnIntegerOverflow=on
  Sum : Sum  Inputs=|++
  u_2 : Outport
  Alpha_2 : Outport  Port=2
  wires:
  Square/1 -> Sum/1
  Square1/1 -> Sum/2
  Sum/1 -> Sqrt/1
  Sqrt/1 -> u_2/1
  u_2x/1 -> Atan2/2, Square/1
  Atan2/1 -> Alpha_2/1
  u_2y/1 -> Atan2/1, Square1/1

== system CSE1_Full/Controller/CtrlCustom_SLX/Controller & Observor/Update law/ellipsoid/ Modified gradient update law ==
  p : Inport
  Us : Inport  Port=2
  p_d : Inport  Port=3
  pd_s : Inport  Port=4
  Divide : Product  Inputs=*/
  Selector : Selector  InputPortWidth=3  IndexOptions=Index vector (dialog)  Indices=[1 2]  OutputSizes=1
  Sum1 : Sum  Inputs=|-+
  "dV/ds  " : MATLAB Function  TreatAsAtomicUnit=on
  length : MATLAB Function  TreatAsAtomicUnit=on
  mu : Gain  Gain=mu  Multiplication=Matrix(K*u)
  s_dot : Outport
  wires:
  mu/1 -> Divide/1
  Divide/1 -> Sum1/1
  "dV/ds  "/1(V_s) -> mu/1
  p_d/1 -> "dV/ds  "/2(p_d)
  pd_s/1 -> "dV/ds  "/3(pd_s), length/1(pd_s)
  length/1(Norm_pd_s) -> Divide/2
  Us/1 -> Sum1/2
  Sum1/1 -> s_dot/1
  p/1 -> Selector/1
  Selector/1 -> "dV/ds  "/1(p)

== system CSE1_Full/Controller/CtrlCustom_SLX/Controller & Observor/Update law/ellipsoid/ellipsoid ==
  s : Inport
  sign : Inport  Port=2
  _ : Constant  Value=Umax_2
  _1 : Constant  Value=center
  _2 : Constant  Value=R
  desired postion path1 : MATLAB Function  TreatAsAtomicUnit=on
  length : MATLAB Function  TreatAsAtomicUnit=on
  Us : Outport
  pd : Outport  Port=2
  pd_s : Outport  Port=3
  pd_ss : Outport  Port=4
  pd_sss : Outport  Port=5
  wires:
  _2/1 -> desired postion path1/2(R)
  _1/1 -> desired postion path1/1(center)
  desired postion path1/1(pd) -> pd/1
  length/1(y) -> Us/1
  s/1 -> desired postion path1/3(s)
  sign/1 -> ?
  desired postion path1/3(pd_ss) -> pd_ss/1
  desired postion path1/4(pd_sss) -> pd_sss/1
  desired postion path1/2(pd_s) -> length/1(pd_s), pd_s/1
  _/1 -> length/2(U_d)

== system CSE1_Full/Controller/CtrlCustom_SLX/Controller & Observor/Update law/ellipsoid/position controller ==
  p : Inport
  pd : Inport  Port=2
  pd_s : Inport  Port=3
  Us : Inport  Port=4
  K : Gain  Gain=diag([0.1,0.1])  Multiplication=Matrix(K*u)
  Product : Product
  Selector : Selector  InputPortWidth=3  IndexOptions=Index vector (dialog)  Indices=[1 2]  OutputSizes=1
  Sum : Sum  Inputs=|+-
  Sum1 : Sum  Inputs=|-+
  u : Outport
  wires:
  Sum/1 -> K/1
  pd_s/1 -> Product/1
  Us/1 -> Product/2
  K/1 -> Sum1/1
  Product/1 -> Sum1/2
  Sum1/1 -> u/1
  pd/1 -> Sum/2
  p/1 -> Selector/1
  Selector/1 -> Sum/1

== system CSE1_Full/Controller/CtrlCustom_SLX/Controller & Observor/Update law/straight line/Unit-tangent gradient update law ==
  p : Inport
  Us : Inport  Port=2
  pd : Inport  Port=3
  pd_s : Inport  Port=4
  Divide : Product  Inputs=*/
  Selector : Selector  InputPortWidth=3  IndexOptions=Index vector (dialog)  Indices=[1 2]  OutputSizes=1
  Sum1 : Sum  Inputs=|-+
  "dV/ds  " : MATLAB Function  TreatAsAtomicUnit=on
  length : MATLAB Function  TreatAsAtomicUnit=on
  mu : Gain  Gain=mu  Multiplication=Matrix(K*u)
  s_dot : Outport
  wires:
  mu/1 -> Divide/1
  Divide/1 -> Sum1/1
  "dV/ds  "/1(V_s) -> mu/1
  pd/1 -> "dV/ds  "/2(pd)
  pd_s/1 -> "dV/ds  "/3(pd_s), length/1(pd_s)
  length/1(Norm_pd_s) -> Divide/2
  Us/1 -> Sum1/2
  Sum1/1 -> s_dot/1
  p/1 -> Selector/1
  Selector/1 -> "dV/ds  "/1(p)

== system CSE1_Full/Controller/CtrlCustom_SLX/Controller & Observor/Update law/straight line/straight line ==
  s : Inport
  eta : Inport  Port=2
  _ : Constant  Value=Umax_1
  _1 : Constant  Value=pd_initial
  _2 : Constant  Value=pd_final
  desired postion path : MATLAB Function  TreatAsAtomicUnit=on
  length : MATLAB Function  TreatAsAtomicUnit=on
  length1 : MATLAB Function  TreatAsAtomicUnit=on
  Us : Outport
  pd : Outport  Port=2
  pd_s : Outport  Port=3
  wires:
  _2/1 -> desired postion path/2(pd_finial)
  _1/1 -> desired postion path/1(pd_initial)
  desired postion path/1(pd) -> pd/1
  desired postion path/2(pd_s) -> length/1(pd_s), pd_s/1
  length/1(y) -> Us/1
  s/1 -> length1/1(s), desired postion path/3(s)
  _/1 -> length1/2(U_max)
  length1/1(U_ref) -> length/2(U_ref)
  eta/1 -> ?

== matlab function CSE1_Full/Simulator CSE1/EquationsOfMotion (Fossen Model)/kinematics ==
  data: nu input; eta_dot output; eta input
function eta_dot = CSE1_eta_dot(nu,eta)

psi = eta(3);

J = [cos(psi) -sin(psi) 0
     sin(psi) cos(psi)  0
     0        0         1];

eta_dot = J*nu;

== matlab function CSE1_Full/Simulator CSE1/EquationsOfMotion (Fossen Model)/kinetics ==
  data: tau input; nu_dot output; nu input
function nu_dot = CSE1_nu_dot(tau,nu)

u   = nu(1);
v   = nu(2);
r   = nu(3);

tau = [tau(1);tau(2);tau(3)];
%% MATRICES 


m    = 14.11;   I_z  =  1.7600;   x_g = 0.0375;       % x_g  =  0.0460; % Table B.1

%% Added mass

X_ud  =     -2.0;											
					Y_vd =      -10.0;	N_vd =    -0.0;		
					Y_rd =      -0.0;	N_rd =    -1.0;		

%% Total mass matrix
m_11 = m-X_ud;
m_22 = m-Y_vd;
m_23 = m*x_g-Y_rd;
m_32 = m*x_g-N_vd; 
m_33 = I_z-N_rd;

M    = [m_11 0    0
        0    m_22 m_23
        0    m_32 m_33];
	
%% Damping coefficients

X_u		= -0.6555;		X_v		= 0;
X_uu 	= 0.3545;		X_vv	= -2.443;
X_uuu 	= -3.787;		X_vvv	= 0;

						Y_v		= -1.33; 			Y_r		= -7.250; 
						Y_vv	= -2.776;			Y_rr	= -3.450; 
						Y_vvv	= -64.91;			Y_rrr	= 0;
						
						Y_rv	= -0.805;			Y_vr	= -0.845; 

						N_v		= 0;				N_r		= -1.900; % N_r
						N_vv	= -0.2088;			N_rr	= -0.750; % N_rr
						N_vvv	= 0;				N_rrr	= 0;
						
						N_rv	= 0.130;			N_vr	= 0.080; % N_rv, N_vr

%% Correolis matrix
c_13 = -(m-Y_vd)*v-(m*x_g-Y_rd)*r;
c_23 = (m-X_ud)*u;
C    = [0     0     c_13
        0     0     c_23
        -c_13 -c_23 0   ];

%% Assembly of the damping matrix
%should be abs(u), abs(v) some places, only positive values? 

d_11 = -X_u - X_uu*u - X_uuu*u^2;
d_22 = -Y_v - Y_vv*v - Y_vvv*v^2 - Y_rv*abs(r);
d_33 = -N_r - N_rr*abs(r) - N_rrr*r^2 - N_vr*abs(v); % using abs(r)

d_12 = -X_v - X_vv*v - X_vvv*v^2;
d_23 = -Y_r - Y_rr*abs(r) - Y_rrr*r^2 - Y_vr*abs(v);
d_32 = -N_v - N_vv*v - N_vvv*v^2 - N_rv*abs(r);


D    = [d_11 0 0
        0    d_22 d_23
        0    d_32 d_33];


%% CALCULATION
nu_dot = M\(tau-(C+D)*nu);

== matlab function CSE1_Full/Controller/CtrlCustom_SLX/Controller & Observor/Update law/straight line/straight line/desired postion path ==
  data: pd_initial input; pd_finial input; pd output; pd_s output; s input size=1
function [pd,pd_s] = fcn(pd_initial,pd_finial,s)

if s >= 1
    s = 1;
end

pd_s = [ (pd_finial(1)-pd_initial(1)); 
                (pd_finial(2)-pd_initial(2))];
% |pd_s| = |pd_p|*|s_dot|

pd =  [(pd_finial(1)-pd_initial(1))*s + pd_initial(1);
        (pd_finial(2)-pd_initial(2))*s + pd_initial(2)];   
end

== matlab function CSE1_Full/Controller/CtrlCustom_SLX/Controller & Observor/Update law/straight line/straight line/length ==
  data: pd_s input; y output; U_ref input
function y = fcn(pd_s,U_ref)

y = U_ref/sqrt(pd_s(1)^2 + pd_s(2)^2);

== matlab function CSE1_Full/Controller/CtrlCustom_SLX/Controller & Observor/Update law/straight line/Unit-tangent gradient update law/dV//ds   ==
  data: p input; V_s output; pd input; pd_s input
function V_s = fcn(p, pd, pd_s)
e = p - pd;
V_s = - transpose(e)*pd_s;

== matlab function CSE1_Full/Controller/CtrlCustom_SLX/Controller & Observor/Update law/straight line/straight line/length1 ==
  data: s input; U_max input; U_ref output
function U_ref = fcn(s, U_max)

if s > 1
    s = 1;
elseif s < 0
    s = 0;
end

U_ref = U_max;

== matlab function CSE1_Full/Controller/CtrlCustom_SLX/Controller & Observor/Update law/straight line/Unit-tangent gradient update law/length ==
  data: pd_s input; Norm_pd_s output
function Norm_pd_s = fcn(pd_s)

Norm_pd_s = sqrt(pd_s(1)^2 + pd_s(2)^2);

== matlab function CSE1_Full/Controller/Switch_function ==
  data: Cross_1 input; switch_signal output; Square_2 input; Circle_3 input; Triangle_4 input; temp input
%% Function that takes in impulse button sigals [0,1] and sends out a 
% different signal depentent pn which button has been pressed

function switch_signal = fcn(Cross_1,Square_2,Circle_3,Triangle_4,temp)
%#codegen
persistent signal;

signal = temp;

if Cross_1 ~= 0
    signal = 1;
end

if Square_2 ~= 0
    signal = 2;
end

if Circle_3 ~= 0
    signal = 3;
end
    
if Triangle_4 ~= 0
    signal = 4; 
end

switch_signal = signal;

== matlab function CSE1_Full/Controller/Sixais Sim ==
  data: Selector input; Out output
%% Function that takes in impulse button sigals [0,1] and sends out a 
% different signal depentent pn which button has been pressed

function Out = fcn(Selector)
%#codegen
if Selector==1
    Out=[1 0 0 0];
elseif Selector==2
        Out=[0 1 0 0];
elseif Selector==4
        Out=[0 0 0 1];
else 
        Out=[0 0 1 0];

end

== matlab function CSE1_Full/Controller/DP_Ctrl/Thrust Allocation /THALOC (u->tau) ==
  data: u input; y output
function y = fcn(u)

y = u;

== matlab function CSE1_Full/Controller/CtrlCustom_SLX/Pose/MATLAB Function ==
  data: angle input; angle output
function angle = rad2pipi(angle)
% RAD2PIPI Converts an angle in rad to the interval <-pi pi>
%          Should be applied to all heading errors in a feedback control system
%          in order to avoid discontinuities.
%
% Author:   Thor I. Fossen
% Date:     21th July June 2001
% Revisions: 

% convert angle in rad to the interval <-pi pi> 
angle = angle - fix(angle/(2*pi))*2*pi;
angle = angle - fix(angle/pi)*2*pi;

== matlab function CSE1_Full/Simulator CSE1/B Command to force mapping/Bow thruster ==
  data: u_BT input; F_y output; nu input
function F_y = fcn(u_BT,nu)
%#codegen
u = nu(1);
% Thruster characteristics
if u_BT >0
    u_BT=u_BT+ 0.059;
    a =        -548;
    b =       0.193;
    c =       548.2;
    d =      0.1992;
    y0 = -(a*exp(b*-u_BT) + c*exp(d*-u_BT));
elseif u_BT < 0
    u_BT=u_BT- 0.059;
    a =        -548;
    b =       0.193;
    c =       548.2;
    d =      0.1992;
    y0 = a*exp(b*u_BT) + c*exp(d*u_BT);
else
    y0 = 0;
end
% Thruster losses due to forward speed
a0 =      0.7561;
a1 =      0.3075;
b1 =      -10.22;
c1 =       2.947;
F_y = y0*(a0 + a1*atan(b1*u +c1))/1.1385;
F_y=F_y*2.62/2.7629;


%2019 changes- Some add-hock changes, because it did not make sense previously.

== matlab function CSE1_Full/Simulator CSE1/B Command to force mapping/VSP ==
  data: alpha input; F_x output; u_VSP input; F_y output
function [ F_x , F_y ] = fcn(alpha,u_VSP)
%#codegen
% Calculating the force in x-direction
a1 =       1.107  ;
b1 =       1.001  ;
c1 =       1.564  ;
a2 =      0.3471 ;
b2 =      0.1397 ;
c2 =      -1.599  ;
a3 =      0.1558 ;
b3 =       1.993  ;
c3 =       1.886  ;
a4 =      0.1599 ;
b4 =       0.218  ;
c4 =       1.513  ;
a5 =     0.08237 ;
b5 =       2.986  ;
c5 =      -1.601  ;
a6 =     0.04641 ;
b6 =       3.964  ;
c6 =       1.738  ;
F_x =   u_VSP*( a1*sin(b1*alpha+c1) + ...
                a2*sin(b2*alpha+c2) + ...
                a3*sin(b3*alpha+c3) + ...
                a4*sin(b4*alpha+c4) + ...
                a5*sin(b5*alpha+c5) + ...
                a6*sin(b6*alpha+c6) );
% Calculating the force in y-direction
a1 =      0.7936 ;
b1 =       1.001  ;
c1 =     0.01605;
a2 =      0.2112 ;
b2 =       1.997  ;
c2 =     0.03229;
a3 =     0.07608;
b3 =       2.991  ;
c3 =       2.986  ;
a4 =     0.04817;
b4 =       3.999  ;
c4 =     -0.8668 ;
a5 =     0.01757;
b5 =       4.904  ;
c5 =      -2.622 ;
a6 =    -0.02089;
b6 =       5.068  ;
c6 =      0.2548 ;
F_y =   u_VSP*( a1*sin(b1*alpha+c1) + ...
                a2*sin(b2*alpha+c2) + ...
                a3*sin(b3*alpha+c3) + ...
                a4*sin(b4*alpha+c4) + ...
                a5*sin(b5*alpha+c5) + ...
                a6*sin(b6*alpha+c6));

== matlab function CSE1_Full/Simulator CSE1/B Command to force mapping/VSP1 ==
  data: alpha input; F_x output; u_VSP input; F_y output
function [ F_x , F_y ] = fcn(alpha,u_VSP)
%#codegen
% Calculating the force in x-direction
a1 =       1.107  ;
b1 =       1.001  ;
c1 =       1.564  ;
a2 =      0.3471 ;
b2 =      0.1397 ;
c2 =      -1.599  ;
a3 =      0.1558 ;
b3 =       1.993  ;
c3 =       1.886  ;
a4 =      0.1599 ;
b4 =       0.218  ;
c4 =       1.513  ;
a5 =     0.08237 ;
b5 =       2.986  ;
c5 =      -1.601  ;
a6 =     0.04641 ;
b6 =       3.964  ;
c6 =       1.738  ;
F_x =   u_VSP*( a1*sin(b1*alpha+c1) + ...
                a2*sin(b2*alpha+c2) + ...
                a3*sin(b3*alpha+c3) + ...
                a4*sin(b4*alpha+c4) + ...
                a5*sin(b5*alpha+c5) + ...
                a6*sin(b6*alpha+c6) );
% Calculating the force in y-direction
a1 =      0.7936 ;
b1 =       1.001  ;
c1 =     0.01605;
a2 =      0.2112 ;
b2 =       1.997  ;
c2 =     0.03229;
a3 =     0.07608;
b3 =       2.991  ;
c3 =       2.986  ;
a4 =     0.04817;
b4 =       3.999  ;
c4 =     -0.8668 ;
a5 =     0.01757;
b5 =       4.904  ;
c5 =      -2.622 ;
a6 =    -0.02089;
b6 =       5.068  ;
c6 =      0.2548 ;
F_y =   u_VSP*( a1*sin(b1*alpha+c1) + ...
                a2*sin(b2*alpha+c2) + ...
                a3*sin(b3*alpha+c3) + ...
                a4*sin(b4*alpha+c4) + ...
                a5*sin(b5*alpha+c5) + ...
                a6*sin(b6*alpha+c6));

== matlab function CSE1_Full/Controller/CtrlCustom_SLX/Controller & Observor/Update law/straight line/MATLAB Function ==
  data: pd input; pd_s input; eta_d output
function eta_d = fcn(pd,pd_s)
%#codegen
psi_d = atan(pd_s(2)/pd_s(1));

eta_d = [pd(1); pd(2); psi_d];

== matlab function CSE1_Full/Controller/CtrlCustom_SLX/Controller & Observor/Update law/straight line/MATLAB Function1 ==
  data: pd_s input; eta_dot output; s_dot input
function eta_dot = fcn(pd_s, s_dot)
eta_dot = [pd_s(1)*s_dot;pd_s(2)*s_dot;0];

== matlab function CSE1_Full/Controller/CtrlCustom_SLX/Controller & Observor/Update law/ellipsoid/ Modified gradient update law/dV//ds   ==
  data: p input; V_s output; p_d input; pd_s input
function V_s = fcn(p, p_d, pd_s)
V_s = - transpose(p - p_d)*pd_s;

== matlab function CSE1_Full/Controller/CtrlCustom_SLX/Controller & Observor/Update law/ellipsoid/ Modified gradient update law/length ==
  data: pd_s input; Norm_pd_s output
function Norm_pd_s = fcn(pd_s)

Norm_pd_s = sqrt(pd_s(1)^2 + pd_s(2)^2);

== matlab function CSE1_Full/Controller/CtrlCustom_SLX/Controller & Observor/Update law/ellipsoid/MATLAB Function ==
  data: pd input; pd_s input; eta_d output
function eta_d = fcn(pd,pd_s)
%#codegen
psi_d = atan(pd_s(2)/pd_s(1));

eta_d = [pd(1); pd(2); psi_d];

== matlab function CSE1_Full/Controller/CtrlCustom_SLX/Controller & Observor/Update law/ellipsoid/MATLAB Function1 ==
  data: pd_s input; eta_dot output; pd_ss input; s_dot input
function eta_dot = fcn(pd_s, pd_ss, s_dot)
%#codegen
psi_d_dot =(pd_s(1)*pd_ss(2)-pd_s(2)*pd_ss(1))/(pd_s(1)^2+ pd_s(2)^2);
eta_dot = [pd_s(1)*s_dot;pd_s(2)*s_dot;psi_d_dot];

== matlab function CSE1_Full/Controller/CtrlCustom_SLX/Controller & Observor/Controller/Controller_parameters/calculating alpha1 ==
  data: z1 input size=[3 1]; K1 input; alpha1 output; eta_d_dot input size=[3 1]; eta_hat input size=[3 1]
function alpha1 = fcn(z1,K1, eta_d_dot, eta_hat)
%#codegen
psi_hat = eta_hat(3);
R = [   cos(psi_hat)    -sin(psi_hat)   0;
        sin(psi_hat)    cos(psi_hat)    0;
        0           0           1;];  

alpha1 = -K1*z1 + transpose(R)*eta_d_dot;

== matlab function CSE1_Full/Controller/CtrlCustom_SLX/Controller & Observor/Update law/ellipsoid/ellipsoid/length ==
  data: pd_s input; y output; U_d input
function y = fcn(pd_s,U_d)

y = U_d/sqrt(pd_s(1)^2 + pd_s(2)^2);

== matlab function CSE1_Full/Controller/CtrlCustom_SLX/Controller & Observor/Controller/Controller_parameters/calculating alpha1_dot ==
  data: z2 input; eta_hat input; nu input size=[3 1]; eta_d_dot input size=[3 1]; K1 input size=[3 3]; alpha1_dot output size=[3 1]; z1 input; eta_d_dot2 input
function alpha1_dot = fcn( z2, eta_hat, nu, eta_d_dot, K1, z1, eta_d_dot2)
%#codegen
r = [0 0 1]*nu;
S = r*[0 -1 0;
     1 0 0;
     0 0 0;];
psi_hat = eta_hat(3);
R = [   cos(psi_hat)    -sin(psi_hat)   0;
        sin(psi_hat)    cos(psi_hat)    0;
        0           0           1;];  

alpha1_dot = K1*(K1+S)*z1 - K1*z2 - S*transpose(R)*eta_d_dot + transpose(R)*eta_d_dot2;

== matlab function CSE1_Full/Controller/CtrlCustom_SLX/Controller & Observor/Update law/ellipsoid/ellipsoid/desired postion path1 ==
  data: center input; R input; pd output; pd_s output; s input size=1; pd_ss output; pd_sss output
function [pd,pd_s, pd_ss, pd_sss] = fcn(center, R, s)

% if s >= 1,
%     s = 1;
% end

pd_sss = [ 8*pi*pi*pi*R(1)*sin(2*pi*s);
           -8*pi*pi*pi*R(2)*cos(2*pi*s)];
       
pd_ss = [ -4*pi*pi*R(1)*cos(2*pi*s);
           -4*pi*pi*R(2)*sin(2*pi*s)];
       
pd_s = [ -2*pi*R(1)*sin(2*pi*s); 
         2*pi*R(2)*cos(2*pi*s)];

pd =  [R(1)*cos(2*pi*s)+center(1);
         R(2)*sin(2*pi*s)+center(2)];   
end

== matlab function CSE1_Full/Controller/CtrlCustom_SLX/Controller & Observor/Update law/ellipsoid/MATLAB Function2 ==
  data: pd_s input; pd_ss input; eta_dot2 output; pd_sss input; s_dot input
function eta_dot2 = fcn(pd_s, pd_ss, pd_sss,s_dot)
%#codegen
psi_d_dot2 =(pd_s(1)*pd_sss(2)-pd_s(2)*pd_sss(1))/(pd_s(1)^2+ pd_s(2)^2)
             - (pd_s(1)*pd_ss(2)-pd_s(2)*pd_ss(1))*(2*pd_s(1)*pd_ss(1)+2*pd_s(2)*pd_ss(2))/(pd_s(1)^2+ pd_s(2)^2)^2;
eta_dot2 = [pd_ss(1)*s_dot;pd_ss(2)*s_dot;psi_d_dot2];

== matlab function CSE1_Full/Controller/CtrlCustom_SLX/Controller & Observor/Controller/Controller_parameters/calculating z1 in BODY-frame ==
  data: eta_d input size=[3 1]; z1 output size=[3 1]; eta_hat input size=[3 1]
function z1 = fcn( eta_d , eta_hat)
%#codegen
psi_hat = eta_hat(3);
R = [   cos(psi_hat)    -sin(psi_hat)   0;
        sin(psi_hat)    cos(psi_hat)    0;
        0           0           1;];  
z1 = transpose(R)*(eta_hat-eta_d);

== matlab function CSE1_Full/Controller/CtrlCustom_SLX/Controller & Observor/Controller/Controller_parameters/calculating z2 ==
  data: alpha1 input size=[3 1]; z2 output size=[3 1]; nu input size=[3 1]
function z2 = fcn( alpha1 , nu)
%#codegen 

z2 = nu-alpha1;

== matlab function CSE1_Full/Controller/CtrlCustom_SLX/Controller & Observor/Controller/MATLAB Function ==
  data: eta_hat input; tau_d output; M input; D input; C input; b input; z1 input; z2 input; alpha1_s input; alpha1 input; K2 input
function tau_d = fcn(eta_hat, M, D, C, b, z1, z2, alpha1_s, alpha1, K2)
%#codegen
psi_hat = eta_hat(3);
R = [   cos(psi_hat)    -sin(psi_hat)   0;
        sin(psi_hat)    cos(psi_hat)    0;
        0           0           0;];  
tau_d = -z1 + (D+C)*alpha1 - transpose(R)*b + M*alpha1_s - K2*z2;

== matlab function CSE1_Full/Controller/CtrlCustom_SLX/Controller & Observor/Controller/MATLAB Function1 ==
  data: nu_hat input; C output
function C = fcn(nu_hat)

u = nu_hat(1);
v = nu_hat(2);
r = nu_hat(3);

m=14.11;
x_g=0.0375;
X_ud=-2;
Y_vd=-10;
Y_rd=0;

C = [ 0             0        (-m*x_g+Y_rd)*r + (-m+Y_vd)*v ;
      0             0        (m-X_ud)*u ;
     (m*x_g-Y_rd)*r + (m-Y_vd)*v    (-m+X_ud)*u      0];
